simulink subsystem "mesh_assembly"  (R2021a)
settings: Solver=VariableStepAuto  StartTime=0.0  StopTime=10.0  RelTol=1e-3
undefined symbols (not defined in the file): dnm, knm, X, Y, Z
libraries: sm_lib x110, mesh_assembly_library x15
(part 2 of 4)

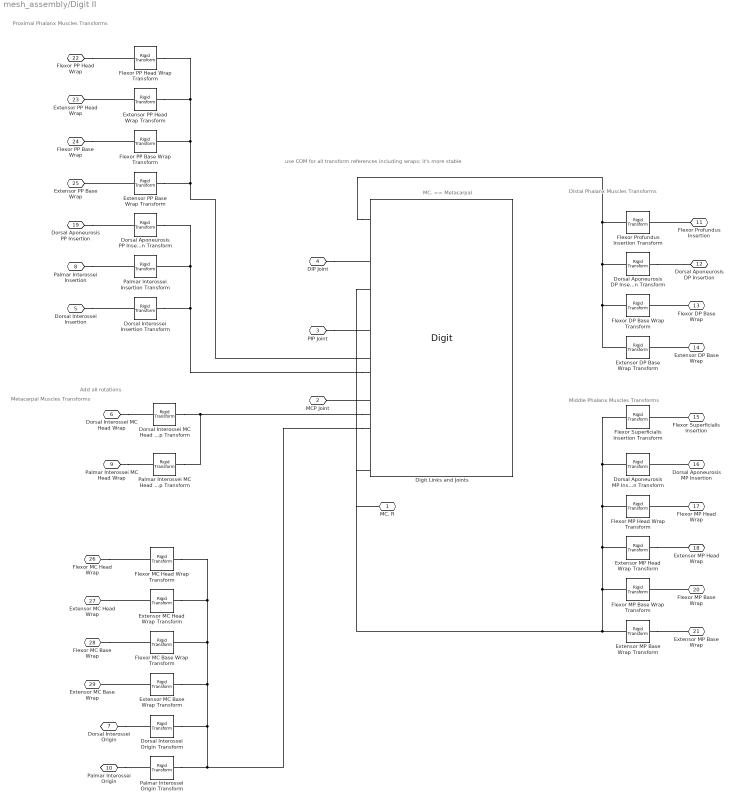
== system mesh_assembly/Digit II ==
  note: MC. == Metacarpal
  note: Proximal Phalanx Muscles Transforms
  note: Distal Phalanx Muscles Transforms
  note: Middle Phalanx Muscles Transforms
  note: Metacarpal Muscles Transforms
  note: Add all rotations
  note: use COM for all transform references including wraps: it's more stable
  Digit Links and Joints : mesh_assembly_library/Digit  links_density=dnm.link_density  distal_phalanx=knm.d2.distal_phalanx.file_name  distal_phalanx_base=knm.d2.distal_phalanx.base_transform  distal_phalanx_dip_joint=knm.d2.distal_phalanx.dip_joint_transform  distal_phalanx_head=knm.d2.distal_phalanx.head_transform  middle_phalanx=knm.d2.middle_phalanx.file_name  middle_phalanx_base=knm.d2.middle_phalanx.base_transform  middle_phalanx_pip_joint=knm.d2.middle_phalanx.pip_joint_transform  middle_phalanx_head=knm.d2.middle_phalanx.head_transform  middle_phalanx_dip_joint=knm.d2.middle_phalanx.dip_joint_transform  proximal_phalanx=knm.d2.proximal_phalanx.file_name  proximal_phalanx_base=knm.d2.proximal_phalanx.base_transform  proximal_phalanx_mcp_joint=knm.d2.proximal_phalanx.mcp_joint_transform  proximal_phalanx_head=knm.d2.proximal_phalanx.head_transform  proximal_phalanx_pip_joint=knm.d2.proximal_phalanx.pip_joint_transform  metacarpal=knm.d2.metacarpal.file_name  metacarpal_base=knm.d2.metacarpal.base_transform  metacarpal_cm_joint=knm.d2.metacarpal.cm_joint_transform  metacarpal_head=knm.d2.metacarpal.head_transform  metacarpal_mcp_joint=knm.d2.metacarpal.mcp_joint_transform  mcp_viz_radius=viz.d2.mcp_joint.radius  mcp_viz_color=viz.d2.mcp_joint.color  mcp_viz_opacity=viz.d2.mcp_joint.opacity  pip_viz_radius=viz.d2.pip_joint.radius  pip_viz_length=viz.d2.pip_joint.length  pip_viz_thickness=viz.d2.pip_joint.thickness  pip_viz_color=viz.d2.pip_joint.color  pip_viz_opacity=viz.d2.pip_joint.opacity  dip_viz_radius=viz.d2.dip_joint.radius  dip_viz_length=viz.d2.dip_joint.length  dip_viz_thickness=viz.d2.dip_joint.thickness  dip_viz_color=viz.d2.dip_joint.color  dip_viz_opacity=viz.d2.dip_joint.opacity
  Dorsal Aponeurosis DP Insertion Transform : sm_lib/Frames and Transforms/Rigid Transform  TranslationMethod=Cartesian  TranslationStandardOffset=0  TranslationLengthUnit=m  TranslationStandardAxis=+Z  TranslationCartesianOffset=knm.d2.distal_phalanx.dorsal_aponeurosis_DP_insertion(1,:)  TranslationROffset=0  TranslationROffsetUnits=m  TranslationZOffset=0  TranslationZOffsetUnits=m  TranslationThetaOffset=0  TranslationThetaOffsetUnits=deg  RotationMethod=RotationSequence  RotationAngleUnits=deg  RotationStandardAxis=+Z  RotationAngle=0.0  RotationArbitraryAxis=[0 0 1]  FollAlignAxisA=+X  BaseAlignAxisA=+Y  FollAlignAxisB=+Y  BaseAlignAxisB=+Z  RotationSequenceAxes=FollowerAxes  RotationSequence=XYZ  RotationSequenceAngles=knm.d2.distal_phalanx.dorsal_aponeurosis_DP_insertion(2,:)  RotationSequenceAnglesUnits=deg  RotationMatrix=[1 0 0; 0 1 0; 0 0 1]
  Dorsal Aponeurosis MP Insertion Transform : sm_lib/Frames and Transforms/Rigid Transform  TranslationMethod=Cartesian  TranslationStandardOffset=0  TranslationLengthUnit=m  TranslationStandardAxis=+Z  TranslationCartesianOffset=knm.d2.middle_phalanx.dorsal_aponeurosis_MP_insertion(1,:)  TranslationROffset=0  TranslationROffsetUnits=m  TranslationZOffset=0  TranslationZOffsetUnits=m  TranslationThetaOffset=0  TranslationThetaOffsetUnits=deg  RotationMethod=RotationSequence  RotationAngleUnits=deg  RotationStandardAxis=+Z  RotationAngle=0.0  RotationArbitraryAxis=[0 0 1]  FollAlignAxisA=+X  BaseAlignAxisA=+Y  FollAlignAxisB=+Y  BaseAlignAxisB=+Z  RotationSequenceAxes=FollowerAxes  RotationSequence=XYZ  RotationSequenceAngles=knm.d2.middle_phalanx.dorsal_aponeurosis_MP_insertion(2,:)  RotationSequenceAnglesUnits=deg  RotationMatrix=[1 0 0; 0 1 0; 0 0 1]
  Dorsal Aponeurosis PP Insertion Transform : sm_lib/Frames and Transforms/Rigid Transform  TranslationMethod=Cartesian  TranslationStandardOffset=0  TranslationLengthUnit=m  TranslationStandardAxis=+Z  TranslationCartesianOffset=knm.d2.proximal_phalanx.dorsal_aponeurosis_PP_insertion(1,:)  TranslationROffset=0  TranslationROffsetUnits=m  TranslationZOffset=0  TranslationZOffsetUnits=m  TranslationThetaOffset=0  TranslationThetaOffsetUnits=deg  RotationMethod=RotationSequence  RotationAngleUnits=deg  RotationStandardAxis=+Z  RotationAngle=0.0  RotationArbitraryAxis=[0 0 1]  FollAlignAxisA=+X  BaseAlignAxisA=+Y  FollAlignAxisB=+Y  BaseAlignAxisB=+Z  RotationSequenceAxes=FollowerAxes  RotationSequence=XYZ  RotationSequenceAngles=knm.d2.proximal_phalanx.dorsal_aponeurosis_PP_insertion(2,:)  RotationSequenceAnglesUnits=deg  RotationMatrix=[1 0 0; 0 1 0; 0 0 1]
  Dorsal Interossei Insertion Transform : sm_lib/Frames and Transforms/Rigid Transform  TranslationMethod=Cartesian  TranslationStandardOffset=0  TranslationLengthUnit=m  TranslationStandardAxis=+Z  TranslationCartesianOffset=knm.d2.proximal_phalanx.dorsal_interossei_insertion_point_transform(1,:)  TranslationROffset=0  TranslationROffsetUnits=m  TranslationZOffset=0  TranslationZOffsetUnits=m  TranslationThetaOffset=0  TranslationThetaOffsetUnits=deg  RotationMethod=RotationSequence  RotationAngleUnits=deg  RotationStandardAxis=+Z  RotationAngle=0.0  RotationArbitraryAxis=[0 0 1]  FollAlignAxisA=+X  BaseAlignAxisA=+Y  FollAlignAxisB=+Y  BaseAlignAxisB=+Z  RotationSequenceAxes=FollowerAxes  RotationSequence=XYZ  RotationSequenceAngles=knm.d2.proximal_phalanx.dorsal_interossei_insertion_point_transform(2,:)  RotationSequenceAnglesUnits=deg  RotationMatrix=[1 0 0; 0 1 0; 0 0 1]
  Dorsal Interossei MC Head Wrap Transform : sm_lib/Frames and Transforms/Rigid Transform  TranslationMethod=Cartesian  TranslationStandardOffset=0  TranslationLengthUnit=m  TranslationStandardAxis=+Z  TranslationCartesianOffset=knm.d2.metacarpal.dorsal_interossei_mc_head_wrap_transform(1,:)  TranslationROffset=0  TranslationROffsetUnits=m  TranslationZOffset=0  TranslationZOffsetUnits=m  TranslationThetaOffset=0  TranslationThetaOffsetUnits=deg  RotationMethod=RotationSequence  RotationAngleUnits=deg  RotationStandardAxis=+Z  RotationAngle=0.0  RotationArbitraryAxis=[0 0 1]  FollAlignAxisA=+X  BaseAlignAxisA=+Y  FollAlignAxisB=+Y  BaseAlignAxisB=+Z  RotationSequenceAxes=FollowerAxes  RotationSequence=XYZ  RotationSequenceAngles=knm.d2.metacarpal.dorsal_interossei_mc_head_wrap_transform(2,:)  RotationSequenceAnglesUnits=deg  RotationMatrix=[1 0 0; 0 1 0; 0 0 1]
  Dorsal Interossei Origin Transform : sm_lib/Frames and Transforms/Rigid Transform  TranslationMethod=Cartesian  TranslationStandardOffset=0  TranslationLengthUnit=m  TranslationStandardAxis=+Z  TranslationCartesianOffset=knm.d2.metacarpal.dorsal_interossei_origin_point_transform(1,:)  TranslationROffset=0  TranslationROffsetUnits=m  TranslationZOffset=0  TranslationZOffsetUnits=m  TranslationThetaOffset=0  TranslationThetaOffsetUnits=deg  RotationMethod=RotationSequence  RotationAngleUnits=deg  RotationStandardAxis=+Z  RotationAngle=0.0  RotationArbitraryAxis=[0 0 1]  FollAlignAxisA=+X  BaseAlignAxisA=+Y  FollAlignAxisB=+Y  BaseAlignAxisB=+Z  RotationSequenceAxes=FollowerAxes  RotationSequence=XYZ  RotationSequenceAngles=knm.d2.metacarpal.dorsal_interossei_origin_point_transform(2,:)  RotationSequenceAnglesUnits=deg  RotationMatrix=[1 0 0; 0 1 0; 0 0 1]
  Extensor DP Base Wrap Transform : sm_lib/Frames and Transforms/Rigid Transform  TranslationMethod=Cartesian  TranslationStandardOffset=0  TranslationLengthUnit=m  TranslationStandardAxis=+Z  TranslationCartesianOffset=knm.d2.distal_phalanx.extensor_base_wrap(1,:)  TranslationROffset=0  TranslationROffsetUnits=m  TranslationZOffset=0  TranslationZOffsetUnits=m  TranslationThetaOffset=0  TranslationThetaOffsetUnits=deg  RotationMethod=RotationSequence  RotationAngleUnits=deg  RotationStandardAxis=+Z  RotationAngle=0.0  RotationArbitraryAxis=[0 0 1]  FollAlignAxisA=+X  BaseAlignAxisA=+Y  FollAlignAxisB=+Y  BaseAlignAxisB=+Z  RotationSequenceAxes=FollowerAxes  RotationSequence=XYZ  RotationSequenceAngles=knm.d2.distal_phalanx.extensor_base_wrap(2,:)  RotationSequenceAnglesUnits=deg  RotationMatrix=[1 0 0; 0 1 0; 0 0 1]
  Extensor MC Base Wrap Transform : sm_lib/Frames and Transforms/Rigid Transform  TranslationMethod=Cartesian  TranslationStandardOffset=0  TranslationLengthUnit=m  TranslationStandardAxis=+Z  TranslationCartesianOffset=knm.d2.metacarpal.extensor_base_wrap(1,:)  TranslationROffset=0  TranslationROffsetUnits=m  TranslationZOffset=0  TranslationZOffsetUnits=m  TranslationThetaOffset=0  TranslationThetaOffsetUnits=deg  RotationMethod=RotationSequence  RotationAngleUnits=deg  RotationStandardAxis=+Z  RotationAngle=0.0  RotationArbitraryAxis=[0 0 1]  FollAlignAxisA=+X  BaseAlignAxisA=+Y  FollAlignAxisB=+Y  BaseAlignAxisB=+Z  RotationSequenceAxes=FollowerAxes  RotationSequence=XYZ  RotationSequenceAngles=knm.d2.metacarpal.extensor_base_wrap(2,:)  RotationSequenceAnglesUnits=deg  RotationMatrix=[1 0 0; 0 1 0; 0 0 1]
  Extensor MC Head Wrap Transform : sm_lib/Frames and Transforms/Rigid Transform  TranslationMethod=Cartesian  TranslationStandardOffset=0  TranslationLengthUnit=m  TranslationStandardAxis=+Z  TranslationCartesianOffset=knm.d2.metacarpal.extensor_head_wrap(1,:)  TranslationROffset=0  TranslationROffsetUnits=m  TranslationZOffset=0  TranslationZOffsetUnits=m  TranslationThetaOffset=0  TranslationThetaOffsetUnits=deg  RotationMethod=RotationSequence  RotationAngleUnits=deg  RotationStandardAxis=+Z  RotationAngle=0.0  RotationArbitraryAxis=[0 0 1]  FollAlignAxisA=+X  BaseAlignAxisA=+Y  FollAlignAxisB=+Y  BaseAlignAxisB=+Z  RotationSequenceAxes=FollowerAxes  RotationSequence=XYZ  RotationSequenceAngles=knm.d2.metacarpal.extensor_head_wrap(2,:)  RotationSequenceAnglesUnits=deg  RotationMatrix=[1 0 0; 0 1 0; 0 0 1]
  Extensor MP Base Wrap Transform : sm_lib/Frames and Transforms/Rigid Transform  TranslationMethod=Cartesian  TranslationStandardOffset=0  TranslationLengthUnit=m  TranslationStandardAxis=+Z  TranslationCartesianOffset=knm.d2.middle_phalanx.extensor_base_wrap(1,:)  TranslationROffset=0  TranslationROffsetUnits=m  TranslationZOffset=0  TranslationZOffsetUnits=m  TranslationThetaOffset=0  TranslationThetaOffsetUnits=deg  RotationMethod=RotationSequence  RotationAngleUnits=deg  RotationStandardAxis=+Z  RotationAngle=0.0  RotationArbitraryAxis=[0 0 1]  FollAlignAxisA=+X  BaseAlignAxisA=+Y  FollAlignAxisB=+Y  BaseAlignAxisB=+Z  RotationSequenceAxes=FollowerAxes  RotationSequence=XYZ  RotationSequenceAngles=knm.d2.middle_phalanx.extensor_base_wrap(2,:)  RotationSequenceAnglesUnits=deg  RotationMatrix=[1 0 0; 0 1 0; 0 0 1]
  Extensor MP Head Wrap Transform : sm_lib/Frames and Transforms/Rigid Transform  TranslationMethod=Cartesian  TranslationStandardOffset=0  TranslationLengthUnit=m  TranslationStandardAxis=+Z  TranslationCartesianOffset=knm.d2.middle_phalanx.extensor_head_wrap(1,:)  TranslationROffset=0  TranslationROffsetUnits=m  TranslationZOffset=0  TranslationZOffsetUnits=m  TranslationThetaOffset=0  TranslationThetaOffsetUnits=deg  RotationMethod=RotationSequence  RotationAngleUnits=deg  RotationStandardAxis=+Z  RotationAngle=0.0  RotationArbitraryAxis=[0 0 1]  FollAlignAxisA=+X  BaseAlignAxisA=+Y  FollAlignAxisB=+Y  BaseAlignAxisB=+Z  RotationSequenceAxes=FollowerAxes  RotationSequence=XYZ  RotationSequenceAngles=knm.d2.middle_phalanx.extensor_head_wrap(2,:)  RotationSequenceAnglesUnits=deg  RotationMatrix=[1 0 0; 0 1 0; 0 0 1]
  Extensor PP Base Wrap Transform : sm_lib/Frames and Transforms/Rigid Transform  TranslationMethod=Cartesian  TranslationStandardOffset=0  TranslationLengthUnit=m  TranslationStandardAxis=+Z  TranslationCartesianOffset=knm.d2.proximal_phalanx.extensor_base_wrap(1,:)  TranslationROffset=0  TranslationROffsetUnits=m  TranslationZOffset=0  TranslationZOffsetUnits=m  TranslationThetaOffset=0  TranslationThetaOffsetUnits=deg  RotationMethod=RotationSequence  RotationAngleUnits=deg  RotationStandardAxis=+Z  RotationAngle=0.0  RotationArbitraryAxis=[0 0 1]  FollAlignAxisA=+X  BaseAlignAxisA=+Y  FollAlignAxisB=+Y  BaseAlignAxisB=+Z  RotationSequenceAxes=FollowerAxes  RotationSequence=XYZ  RotationSequenceAngles=knm.d2.proximal_phalanx.extensor_base_wrap(2,:)  RotationSequenceAnglesUnits=deg  RotationMatrix=[1 0 0; 0 1 0; 0 0 1]
  Extensor PP Head Wrap Transform : sm_lib/Frames and Transforms/Rigid Transform  TranslationMethod=Cartesian  TranslationStandardOffset=0  TranslationLengthUnit=m  TranslationStandardAxis=+Z  TranslationCartesianOffset=knm.d2.proximal_phalanx.extensor_head_wrap(1,:)  TranslationROffset=0  TranslationROffsetUnits=m  TranslationZOffset=0  TranslationZOffsetUnits=m  TranslationThetaOffset=0  TranslationThetaOffsetUnits=deg  RotationMethod=RotationSequence  RotationAngleUnits=deg  RotationStandardAxis=+Z  RotationAngle=0.0  RotationArbitraryAxis=[0 0 1]  FollAlignAxisA=+X  BaseAlignAxisA=+Y  FollAlignAxisB=+Y  BaseAlignAxisB=+Z  RotationSequenceAxes=FollowerAxes  RotationSequence=XYZ  RotationSequenceAngles=knm.d2.proximal_phalanx.extensor_head_wrap(2,:)  RotationSequenceAnglesUnits=deg  RotationMatrix=[1 0 0; 0 1 0; 0 0 1]
  Flexor DP Base Wrap Transform : sm_lib/Frames and Transforms/Rigid Transform  TranslationMethod=Cartesian  TranslationStandardOffset=0  TranslationLengthUnit=m  TranslationStandardAxis=+Z  TranslationCartesianOffset=knm.d2.distal_phalanx.flexor_base_wrap(1,:)  TranslationROffset=0  TranslationROffsetUnits=m  TranslationZOffset=0  TranslationZOffsetUnits=m  TranslationThetaOffset=0  TranslationThetaOffsetUnits=deg  RotationMethod=RotationSequence  RotationAngleUnits=deg  RotationStandardAxis=+Z  RotationAngle=0.0  RotationArbitraryAxis=[0 0 1]  FollAlignAxisA=+X  BaseAlignAxisA=+Y  FollAlignAxisB=+Y  BaseAlignAxisB=+Z  RotationSequenceAxes=FollowerAxes  RotationSequence=XYZ  RotationSequenceAngles=knm.d2.distal_phalanx.flexor_base_wrap(2,:)  RotationSequenceAnglesUnits=deg  RotationMatrix=[1 0 0; 0 1 0; 0 0 1]
  Flexor MC Base Wrap Transform : sm_lib/Frames and Transforms/Rigid Transform  TranslationMethod=Cartesian  TranslationStandardOffset=0  TranslationLengthUnit=m  TranslationStandardAxis=+Z  TranslationCartesianOffset=knm.d2.metacarpal.flexor_base_wrap(1,:)  TranslationROffset=0  TranslationROffsetUnits=m  TranslationZOffset=0  TranslationZOffsetUnits=m  TranslationThetaOffset=0  TranslationThetaOffsetUnits=deg  RotationMethod=RotationSequence  RotationAngleUnits=deg  RotationStandardAxis=+Z  RotationAngle=0.0  RotationArbitraryAxis=[0 0 1]  FollAlignAxisA=+X  BaseAlignAxisA=+Y  FollAlignAxisB=+Y  BaseAlignAxisB=+Z  RotationSequenceAxes=FollowerAxes  RotationSequence=XYZ  RotationSequenceAngles=knm.d2.metacarpal.flexor_base_wrap(2,:)  RotationSequenceAnglesUnits=deg  RotationMatrix=[1 0 0; 0 1 0; 0 0 1]
  Flexor MC Head Wrap Transform : sm_lib/Frames and Transforms/Rigid Transform  TranslationMethod=Cartesian  TranslationStandardOffset=0  TranslationLengthUnit=m  TranslationStandardAxis=+Z  TranslationCartesianOffset=knm.d2.metacarpal.flexor_head_wrap(1,:)  TranslationROffset=0  TranslationROffsetUnits=m  TranslationZOffset=0  TranslationZOffsetUnits=m  TranslationThetaOffset=0  TranslationThetaOffsetUnits=deg  RotationMethod=RotationSequence  RotationAngleUnits=deg  RotationStandardAxis=+Z  RotationAngle=0.0  RotationArbitraryAxis=[0 0 1]  FollAlignAxisA=+X  BaseAlignAxisA=+Y  FollAlignAxisB=+Y  BaseAlignAxisB=+Z  RotationSequenceAxes=FollowerAxes  RotationSequence=XYZ  RotationSequenceAngles=knm.d2.metacarpal.flexor_head_wrap(2,:)  RotationSequenceAnglesUnits=deg  RotationMatrix=[1 0 0; 0 1 0; 0 0 1]
  Flexor MP Base Wrap Transform : sm_lib/Frames and Transforms/Rigid Transform  TranslationMethod=Cartesian  TranslationStandardOffset=0  TranslationLengthUnit=m  TranslationStandardAxis=+Z  TranslationCartesianOffset=knm.d2.middle_phalanx.flexor_base_wrap(1,:)  TranslationROffset=0  TranslationROffsetUnits=m  TranslationZOffset=0  TranslationZOffsetUnits=m  TranslationThetaOffset=0  TranslationThetaOffsetUnits=deg  RotationMethod=RotationSequence  RotationAngleUnits=deg  RotationStandardAxis=+Z  RotationAngle=0.0  RotationArbitraryAxis=[0 0 1]  FollAlignAxisA=+X  BaseAlignAxisA=+Y  FollAlignAxisB=+Y  BaseAlignAxisB=+Z  RotationSequenceAxes=FollowerAxes  RotationSequence=XYZ  RotationSequenceAngles=knm.d2.middle_phalanx.flexor_base_wrap(2,:)  RotationSequenceAnglesUnits=deg  RotationMatrix=[1 0 0; 0 1 0; 0 0 1]
  Flexor MP Head Wrap Transform : sm_lib/Frames and Transforms/Rigid Transform  TranslationMethod=Cartesian  TranslationStandardOffset=0  TranslationLengthUnit=m  TranslationStandardAxis=+Z  TranslationCartesianOffset=knm.d2.middle_phalanx.flexor_head_wrap(1,:)  TranslationROffset=0  TranslationROffsetUnits=m  TranslationZOffset=0  TranslationZOffsetUnits=m  TranslationThetaOffset=0  TranslationThetaOffsetUnits=deg  RotationMethod=RotationSequence  RotationAngleUnits=deg  RotationStandardAxis=+Z  RotationAngle=0.0  RotationArbitraryAxis=[0 0 1]  FollAlignAxisA=+X  BaseAlignAxisA=+Y  FollAlignAxisB=+Y  BaseAlignAxisB=+Z  RotationSequenceAxes=FollowerAxes  RotationSequence=XYZ  RotationSequenceAngles=knm.d2.middle_phalanx.flexor_head_wrap(2,:)  RotationSequenceAnglesUnits=deg  RotationMatrix=[1 0 0; 0 1 0; 0 0 1]
  Flexor PP Base Wrap Transform : sm_lib/Frames and Transforms/Rigid Transform  TranslationMethod=Cartesian  TranslationStandardOffset=0  TranslationLengthUnit=m  TranslationStandardAxis=+Z  TranslationCartesianOffset=knm.d2.proximal_phalanx.flexor_base_wrap(1,:)  TranslationROffset=0  TranslationROffsetUnits=m  TranslationZOffset=0  TranslationZOffsetUnits=m  TranslationThetaOffset=0  TranslationThetaOffsetUnits=deg  RotationMethod=RotationSequence  RotationAngleUnits=deg  RotationStandardAxis=+Z  RotationAngle=0.0  RotationArbitraryAxis=[0 0 1]  FollAlignAxisA=+X  BaseAlignAxisA=+Y  FollAlignAxisB=+Y  BaseAlignAxisB=+Z  RotationSequenceAxes=FollowerAxes  RotationSequence=XYZ  RotationSequenceAngles=knm.d2.proximal_phalanx.flexor_base_wrap(2,:)  RotationSequenceAnglesUnits=deg  RotationMatrix=[1 0 0; 0 1 0; 0 0 1]
  Flexor PP Head Wrap Transform : sm_lib/Frames and Transforms/Rigid Transform  TranslationMethod=Cartesian  TranslationStandardOffset=0  TranslationLengthUnit=m  TranslationStandardAxis=+Z  TranslationCartesianOffset=knm.d2.proximal_phalanx.flexor_head_wrap(1,:)  TranslationROffset=0  TranslationROffsetUnits=m  TranslationZOffset=0  TranslationZOffsetUnits=m  TranslationThetaOffset=0  TranslationThetaOffsetUnits=deg  RotationMethod=RotationSequence  RotationAngleUnits=deg  RotationStandardAxis=+Z  RotationAngle=0.0  RotationArbitraryAxis=[0 0 1]  FollAlignAxisA=+X  BaseAlignAxisA=+Y  FollAlignAxisB=+Y  BaseAlignAxisB=+Z  RotationSequenceAxes=FollowerAxes  RotationSequence=XYZ  RotationSequenceAngles=knm.d2.proximal_phalanx.flexor_head_wrap(2,:)  RotationSequenceAnglesUnits=deg  RotationMatrix=[1 0 0; 0 1 0; 0 0 1]
  Flexor Profundus Insertion Transform : sm_lib/Frames and Transforms/Rigid Transform  TranslationMethod=Cartesian  TranslationStandardOffset=0  TranslationLengthUnit=m  TranslationStandardAxis=+Z  TranslationCartesianOffset=knm.d2.distal_phalanx.flexor_profundus_insertion(1,:)  TranslationROffset=0  TranslationROffsetUnits=m  TranslationZOffset=0  TranslationZOffsetUnits=m  TranslationThetaOffset=0  TranslationThetaOffsetUnits=deg  RotationMethod=RotationSequence  RotationAngleUnits=deg  RotationStandardAxis=+Z  RotationAngle=0.0  RotationArbitraryAxis=[0 0 1]  FollAlignAxisA=+X  BaseAlignAxisA=+Y  FollAlignAxisB=+Y  BaseAlignAxisB=+Z  RotationSequenceAxes=FollowerAxes  RotationSequence=XYZ  RotationSequenceAngles=knm.d2.distal_phalanx.flexor_profundus_insertion(2,:)  RotationSequenceAnglesUnits=deg  RotationMatrix=[1 0 0; 0 1 0; 0 0 1]
  Flexor Superficialis Insertion Transform : sm_lib/Frames and Transforms/Rigid Transform  TranslationMethod=Cartesian  TranslationStandardOffset=0  TranslationLengthUnit=m  TranslationStandardAxis=+Z  TranslationCartesianOffset=knm.d2.middle_phalanx.flexor_superficialis_insertion(1,:)  TranslationROffset=0  TranslationROffsetUnits=m  TranslationZOffset=0  TranslationZOffsetUnits=m  TranslationThetaOffset=0  TranslationThetaOffsetUnits=deg  RotationMethod=RotationSequence  RotationAngleUnits=deg  RotationStandardAxis=+Z  RotationAngle=0.0  RotationArbitraryAxis=[0 0 1]  FollAlignAxisA=+X  BaseAlignAxisA=+Y  FollAlignAxisB=+Y  BaseAlignAxisB=+Z  RotationSequenceAxes=FollowerAxes  RotationSequence=XYZ  RotationSequenceAngles=knm.d2.middle_phalanx.flexor_superficialis_insertion(2,:)  RotationSequenceAnglesUnits=deg  RotationMatrix=[1 0 0; 0 1 0; 0 0 1]
  Palmar Interossei Insertion Transform : sm_lib/Frames and Transforms/Rigid Transform  TranslationMethod=Cartesian  TranslationStandardOffset=0  TranslationLengthUnit=m  TranslationStandardAxis=+Z  TranslationCartesianOffset=knm.d2.proximal_phalanx.palmar_interossei_insertion_point_transform(1,:)  TranslationROffset=0  TranslationROffsetUnits=m  TranslationZOffset=0  TranslationZOffsetUnits=m  TranslationThetaOffset=0  TranslationThetaOffsetUnits=deg  RotationMethod=RotationSequence  RotationAngleUnits=deg  RotationStandardAxis=+Z  RotationAngle=0.0  RotationArbitraryAxis=[0 0 1]  FollAlignAxisA=+X  BaseAlignAxisA=+Y  FollAlignAxisB=+Y  BaseAlignAxisB=+Z  RotationSequenceAxes=FollowerAxes  RotationSequence=XYZ  RotationSequenceAngles=knm.d2.proximal_phalanx.palmar_interossei_insertion_point_transform(2,:)  RotationSequenceAnglesUnits=deg  RotationMatrix=[1 0 0; 0 1 0; 0 0 1]
  Palmar Interossei MC Head Wrap Transform : sm_lib/Frames and Transforms/Rigid Transform  TranslationMethod=Cartesian  TranslationStandardOffset=0  TranslationLengthUnit=m  TranslationStandardAxis=+Z  TranslationCartesianOffset=knm.d2.metacarpal.palmar_interossei_mc_head_wrap_transform(1,:)  TranslationROffset=0  TranslationROffsetUnits=m  TranslationZOffset=0  TranslationZOffsetUnits=m  TranslationThetaOffset=0  TranslationThetaOffsetUnits=deg  RotationMethod=RotationSequence  RotationAngleUnits=deg  RotationStandardAxis=+Z  RotationAngle=0.0  RotationArbitraryAxis=[0 0 1]  FollAlignAxisA=+X  BaseAlignAxisA=+Y  FollAlignAxisB=+Y  BaseAlignAxisB=+Z  RotationSequenceAxes=FollowerAxes  RotationSequence=XYZ  RotationSequenceAngles=knm.d2.metacarpal.palmar_interossei_mc_head_wrap_transform(2,:)  RotationSequenceAnglesUnits=deg  RotationMatrix=[1 0 0; 0 1 0; 0 0 1]
  Palmar Interossei Origin Transform : sm_lib/Frames and Transforms/Rigid Transform  TranslationMethod=Cartesian  TranslationStandardOffset=0  TranslationLengthUnit=m  TranslationStandardAxis=+Z  TranslationCartesianOffset=knm.d2.metacarpal.palmar_interossei_origin_point_transform(1,:)  TranslationROffset=0  TranslationROffsetUnits=m  TranslationZOffset=0  TranslationZOffsetUnits=m  TranslationThetaOffset=0  TranslationThetaOffsetUnits=deg  RotationMethod=RotationSequence  RotationAngleUnits=deg  RotationStandardAxis=+Z  RotationAngle=0.0  RotationArbitraryAxis=[0 0 1]  FollAlignAxisA=+X  BaseAlignAxisA=+Y  FollAlignAxisB=+Y  BaseAlignAxisB=+Z  RotationSequenceAxes=FollowerAxes  RotationSequence=XYZ  RotationSequenceAngles=knm.d2.metacarpal.palmar_interossei_origin_point_transform(2,:)  RotationSequenceAnglesUnits=deg  RotationMatrix=[1 0 0; 0 1 0; 0 0 1]
  MC. R : PMIOPort  Side=Left
  MCP Joint : PMIOPort  Port=2  Side=Left
  PIP Joint : PMIOPort  Port=3  Side=Left
  DIP Joint : PMIOPort  Port=4  Side=Left
  Dorsal Interossei Insertion : PMIOPort  Port=5  Side=Left
  Dorsal Interossei MC Head Wrap : PMIOPort  Port=6  Side=Left
  Dorsal Interossei Origin : PMIOPort  Port=7  Side=Left
  Palmar Interossei Insertion : PMIOPort  Port=8  Side=Left
  Palmar Interossei MC Head Wrap : PMIOPort  Port=9  Side=Left
  Palmar Interossei Origin : PMIOPort  Port=10  Side=Left
  Flexor Profundus Insertion : PMIOPort  Port=11  Side=Left
  Dorsal Aponeurosis DP Insertion : PMIOPort  Port=12  Side=Left
  Flexor DP Base Wrap : PMIOPort  Port=13  Side=Left
  Extensor DP Base Wrap : PMIOPort  Port=14  Side=Left
  Flexor Superficialis Insertion : PMIOPort  Port=15  Side=Left
  Dorsal Aponeurosis MP Insertion : PMIOPort  Port=16  Side=Left
  Flexor MP Head Wrap : PMIOPort  Port=17  Side=Left
  Extensor MP Head Wrap : PMIOPort  Port=18  Side=Left
  Dorsal Aponeurosis PP Insertion : PMIOPort  Port=19  Side=Left
  Flexor MP Base Wrap : PMIOPort  Port=20  Side=Left
  Extensor MP Base Wrap : PMIOPort  Port=21  Side=Left
  Flexor PP Head Wrap : PMIOPort  Port=22  Side=Left
  Extensor PP Head Wrap : PMIOPort  Port=23  Side=Left
  Flexor PP Base Wrap : PMIOPort  Port=24  Side=Left
  Extensor PP Base Wrap : PMIOPort  Port=25  Side=Left
  Flexor MC Head Wrap : PMIOPort  Port=26  Side=Left
  Extensor MC Head Wrap : PMIOPort  Port=27  Side=Left
  Flexor MC Base Wrap : PMIOPort  Port=28  Side=Left
  Extensor MC Base Wrap : PMIOPort  Port=29  Side=Left
  connections:
  Extensor MC Base Wrap Transform/RConn1 -- Extensor MC Base Wrap/RConn1
  Flexor MC Base Wrap/RConn1 -- Flexor MC Base Wrap Transform/RConn1
  Flexor MC Head Wrap/RConn1 -- Flexor MC Head Wrap Transform/RConn1
  Extensor MC Head Wrap Transform/RConn1 -- Extensor MC Head Wrap/RConn1
  Digit Links and Joints/LConn17 -- Palmar Interossei Origin Transform/LConn1 -- Dorsal Interossei Origin Transform/LConn1 -- Extensor MC Base Wrap Transform/LConn1 -- Flexor MC Head Wrap Transform/LConn1 -- Extensor MC Head Wrap Transform/LConn1 -- Flexor MC Base Wrap Transform/LConn1
  Digit Links and Joints/LConn12 -- Extensor PP Base Wrap Transform/LConn1 -- Flexor PP Base Wrap Transform/LConn1 -- Extensor PP Head Wrap Transform/LConn1 -- Flexor PP Head Wrap Transform/LConn1
  Extensor PP Head Wrap Transform/RConn1 -- Extensor PP Head Wrap/RConn1
  Flexor PP Head Wrap/RConn1 -- Flexor PP Head Wrap Transform/RConn1
  Flexor PP Base Wrap/RConn1 -- Flexor PP Base Wrap Transform/RConn1
  Extensor PP Base Wrap Transform/RConn1 -- Extensor PP Base Wrap/RConn1
  Digit Links and Joints/LConn13 -- Palmar Interossei Insertion Transform/LConn1 -- Dorsal Aponeurosis PP Insertion Transform/LConn1 -- Dorsal Interossei Insertion Transform/LConn1
  Flexor MP Base Wrap/RConn1 -- Flexor MP Base Wrap Transform/RConn1
  Extensor MP Base Wrap Transform/RConn1 -- Extensor MP Base Wrap/RConn1
  Dorsal Aponeurosis PP Insertion/RConn1 -- Dorsal Aponeurosis PP Insertion Transform/RConn1
  Extensor MP Head Wrap Transform/RConn1 -- Extensor MP Head Wrap/RConn1
  Flexor MP Head Wrap/RConn1 -- Flexor MP Head Wrap Transform/RConn1
  Dorsal Aponeurosis MP Insertion/RConn1 -- Dorsal Aponeurosis MP Insertion Transform/RConn1
  Flexor Superficialis Insertion/RConn1 -- Flexor Superficialis Insertion Transform/RConn1
  Dorsal Aponeurosis DP Insertion Transform/RConn1 -- Dorsal Aponeurosis DP Insertion/RConn1
  Flexor DP Base Wrap/RConn1 -- Flexor DP Base Wrap Transform/RConn1
  Extensor DP Base Wrap/RConn1 -- Extensor DP Base Wrap Transform/RConn1
  Flexor Profundus Insertion/RConn1 -- Flexor Profundus Insertion Transform/RConn1
  Digit Links and Joints/LConn2 -- Dorsal Aponeurosis DP Insertion Transform/LConn1 -- Flexor DP Base Wrap Transform/LConn1 -- Extensor DP Base Wrap Transform/LConn1 -- Flexor Profundus Insertion Transform/LConn1
  Digit Links and Joints/LConn7 -- Extensor MP Base Wrap Transform/LConn1 -- Flexor MP Base Wrap Transform/LConn1 -- Extensor MP Head Wrap Transform/LConn1 -- Flexor MP Head Wrap Transform/LConn1 -- Dorsal Aponeurosis MP Insertion Transform/LConn1 -- Flexor Superficialis Insertion Transform/LConn1
  Palmar Interossei Insertion/RConn1 -- Palmar Interossei Insertion Transform/RConn1
  Palmar Interossei MC Head Wrap/RConn1 -- Palmar Interossei MC Head Wrap Transform/RConn1
  Palmar Interossei Origin/RConn1 -- Palmar Interossei Origin Transform/RConn1
  Dorsal Interossei Origin/RConn1 -- Dorsal Interossei Origin Transform/RConn1
  Dorsal Interossei MC Head Wrap/RConn1 -- Dorsal Interossei MC Head Wrap Transform/RConn1
  Dorsal Interossei Insertion/RConn1 -- Dorsal Interossei Insertion Transform/RConn1
  Digit Links and Joints/LConn16 -- Dorsal Interossei MC Head Wrap Transform/LConn1 -- Palmar Interossei MC Head Wrap Transform/LConn1
  DIP Joint/RConn1 -- Digit Links and Joints/LConn5
  PIP Joint/RConn1 -- Digit Links and Joints/LConn10
  Digit Links and Joints/LConn15 -- MCP Joint/RConn1
  MC. R/RConn1 -- Digit Links and Joints/LConn20

== system mesh_assembly/Digit III ==
  note: MC. == Metacarpal
  Digit Links and Joints : Subsystem  AncestorBlock=mechanics_model_library/Digit  mask{links_density=dnm.link_density, distal_phalanx=knm.d3.distal_phalanx.file_name, distal_phalanx_base=knm.d3.distal_phalanx.base_transform, distal_phalanx_dip_joint=knm.d3.distal_phalanx.dip_joint_transform, distal_phalanx_head=knm.d3.distal_phalanx.head_transform, middle_phalanx=knm.d3.middle_phalanx.file_name, middle_phalanx_base=knm.d3.middle_phalanx.base_transform, middle_phalanx_pip_joint=knm.d3.middle_phalanx.pip_joint_transform, middle_phalanx_head=knm.d3.middle_phalanx.head_transform, middle_phalanx_dip_joint=knm.d3.middle_phalanx.dip_joint_transform, proximal_phalanx=knm.d3.proximal_phalanx.file_name, proximal_phalanx_base=knm.d3.proximal_phalanx.base_transform, proximal_phalanx_mcp_joint=knm.d3.proximal_phalanx.mcp_joint_transform, proximal_phalanx_head=knm.d3.proximal_phalanx.head_transform, proximal_phalanx_pip_joint=knm.d3.proximal_phalanx.pip_joint_transform, metacarpal=knm.d3.metacarpal.file_name, metacarpal_base=knm.d3.metacarpal.base_transform, metacarpal_cm_joint=knm.d3.metacarpal.cm_joint_transform, metacarpal_head=knm.d3.metacarpal.head_transform, metacarpal_mcp_joint=knm.d3.metacarpal.mcp_joint_transform, mcp_viz_radius=viz.d3.mcp_joint.radius, mcp_viz_color=viz.d3.mcp_joint.color, mcp_viz_opacity=viz.d3.mcp_joint.opacity, pip_viz_radius=viz.d3.pip_joint.radius, pip_viz_length=viz.d3.pip_joint.length, pip_viz_thickness=viz.d3.pip_joint.thickness, pip_viz_color=viz.d3.pip_joint.color, pip_viz_opacity=viz.d3.pip_joint.opacity, dip_viz_radius=viz.d3.dip_joint.radius, dip_viz_length=viz.d3.dip_joint.length, dip_viz_thickness=viz.d3.dip_joint.thickness, dip_viz_color=viz.d3.dip_joint.color, dip_viz_opacity=viz.d3.dip_joint.opacity}
      mask prompts: links_density "Density [Kg/(m^3)]"; distal_phalanx "File Name"; distal_phalanx_base "Base Transform (Translation [m], Rotation: X-Y-Z [deg])"; distal_phalanx_dip_joint "DIP Joint Transform (Translation, Rotation)"; distal_phalanx_head "Head Transform (Translation, Rotation)"; middle_phalanx "File Name"; middle_phalanx_base "Base Transform"; middle_phalanx_pip_joint "PIP Joint Transform"; middle_phalanx_head "Head Transform"; middle_phalanx_dip_joint "DIP Joint Transform"; proximal_phalanx "File Name"; proximal_phalanx_base "Base Transform"; proximal_phalanx_mcp_joint "MCP Joint Transform"; proximal_phalanx_head "Head Transform"; proximal_phalanx_pip_joint "PIP Joint Transform"; metacarpal "File Name"; metacarpal_base "Base Transform"; metacarpal_cm_joint "CM Joint Transform"; metacarpal_head "Head Transform"; metacarpal_mcp_joint "MCP Joint Transform"; mcp_viz_radius "Radius [m]"; mcp_viz_color "Color (RGB - Range [0, 1])"; mcp_viz_opacity "Opacity (Range [0, 1])"; pip_viz_radius "Radius [m]"; pip_viz_length "Length [m]"; pip_viz_thickness "Thickness [m]"; pip_viz_color "Color (RGB - Range [0, 1])"; pip_viz_opacity "Opacity (Range [0, 1])"; dip_viz_radius "Radius [m]"; dip_viz_length "Length [m]"; dip_viz_thickness "Thickness [m]"; dip_viz_color "Color (RGB - Range [0, 1])"; dip_viz_opacity "Opacity (Range [0, 1])"
      mask DialogControl DescGroupVar Prompt: Digit Subsystem
      mask DialogControl DescTextVar Prompt: This subsystem encapsulates the bones and joints that makes up digits II - V. Metacarpal bone, Proximal, Middle and Distal Phalanxes; MCP, PIP and DIP Joints.
      mask DialogControl Links Prompt: Links
      mask DialogControl Distal_Phalanx Prompt: Distal Phalanx
      mask DialogControl Middle_Phalanx Prompt: Middle Phalanx
      mask DialogControl Proximal_Phalanx Prompt: Proximal Phalanx
      mask DialogControl Metacarpal Prompt: Metacarpal
      mask DialogControl Container10 Prompt: Visualization
      mask DialogControl Container11 Prompt: MCP Joint
      mask DialogControl Container12 Prompt: PIP Joint
      mask DialogControl Container13 Prompt: DIP Joint
  MC. R : PMIOPort  Side=Left
  MCP Joint : PMIOPort  Port=2  Side=Left
  PIP Joint : PMIOPort  Port=3  Side=Left
  DIP Joint : PMIOPort  Port=4  Side=Left
  connections:
  PIP Joint/RConn1 -- Digit Links and Joints/LConn10
  Digit Links and Joints/LConn15 -- MCP Joint/RConn1
  MC. R/RConn1 -- Digit Links and Joints/LConn20
  DIP Joint/RConn1 -- Digit Links and Joints/LConn5

== system mesh_assembly/Digit IV ==
  note: MC. == Metacarpal
  Digit Links and Joints : Subsystem  AncestorBlock=mechanics_model_library/Digit  mask{links_density=dnm.link_density, distal_phalanx=knm.d4.distal_phalanx.file_name, distal_phalanx_base=knm.d4.distal_phalanx.base_transform, distal_phalanx_dip_joint=knm.d4.distal_phalanx.dip_joint_transform, distal_phalanx_head=knm.d4.distal_phalanx.head_transform, middle_phalanx=knm.d4.middle_phalanx.file_name, middle_phalanx_base=knm.d4.middle_phalanx.base_transform, middle_phalanx_pip_joint=knm.d4.middle_phalanx.pip_joint_transform, middle_phalanx_head=knm.d4.middle_phalanx.head_transform, middle_phalanx_dip_joint=knm.d4.middle_phalanx.dip_joint_transform, proximal_phalanx=knm.d4.proximal_phalanx.file_name, proximal_phalanx_base=knm.d4.proximal_phalanx.base_transform, proximal_phalanx_mcp_joint=knm.d4.proximal_phalanx.mcp_joint_transform, proximal_phalanx_head=knm.d4.proximal_phalanx.head_transform, proximal_phalanx_pip_joint=knm.d4.proximal_phalanx.pip_joint_transform, metacarpal=knm.d4.metacarpal.file_name, metacarpal_base=knm.d4.metacarpal.base_transform, metacarpal_cm_joint=knm.d4.metacarpal.cm_joint_transform, metacarpal_head=knm.d4.metacarpal.head_transform, metacarpal_mcp_joint=knm.d4.metacarpal.mcp_joint_transform, mcp_viz_radius=viz.d4.mcp_joint.radius, mcp_viz_color=viz.d4.mcp_joint.color, mcp_viz_opacity=viz.d4.mcp_joint.opacity, pip_viz_radius=viz.d4.pip_joint.radius, pip_viz_length=viz.d4.pip_joint.length, pip_viz_thickness=viz.d4.pip_joint.thickness, pip_viz_color=viz.d4.pip_joint.color, pip_viz_opacity=viz.d4.pip_joint.opacity, dip_viz_radius=viz.d4.dip_joint.radius, dip_viz_length=viz.d4.dip_joint.length, dip_viz_thickness=viz.d4.dip_joint.thickness, dip_viz_color=viz.d4.dip_joint.color, dip_viz_opacity=viz.d4.dip_joint.opacity}
      mask prompts: links_density "Density [Kg/(m^3)]"; distal_phalanx "File Name"; distal_phalanx_base "Base Transform (Translation [m], Rotation: X-Y-Z [deg])"; distal_phalanx_dip_joint "DIP Joint Transform (Translation, Rotation)"; distal_phalanx_head "Head Transform (Translation, Rotation)"; middle_phalanx "File Name"; middle_phalanx_base "Base Transform"; middle_phalanx_pip_joint "PIP Joint Transform"; middle_phalanx_head "Head Transform"; middle_phalanx_dip_joint "DIP Joint Transform"; proximal_phalanx "File Name"; proximal_phalanx_base "Base Transform"; proximal_phalanx_mcp_joint "MCP Joint Transform"; proximal_phalanx_head "Head Transform"; proximal_phalanx_pip_joint "PIP Joint Transform"; metacarpal "File Name"; metacarpal_base "Base Transform"; metacarpal_cm_joint "CM Joint Transform"; metacarpal_head "Head Transform"; metacarpal_mcp_joint "MCP Joint Transform"; mcp_viz_radius "Radius [m]"; mcp_viz_color "Color (RGB - Range [0, 1])"; mcp_viz_opacity "Opacity (Range [0, 1])"; pip_viz_radius "Radius [m]"; pip_viz_length "Length [m]"; pip_viz_thickness "Thickness [m]"; pip_viz_color "Color (RGB - Range [0, 1])"; pip_viz_opacity "Opacity (Range [0, 1])"; dip_viz_radius "Radius [m]"; dip_viz_length "Length [m]"; dip_viz_thickness "Thickness [m]"; dip_viz_color "Color (RGB - Range [0, 1])"; dip_viz_opacity "Opacity (Range [0, 1])"
      mask DialogControl DescGroupVar Prompt: Digit Subsystem
      mask DialogControl DescTextVar Prompt: This subsystem encapsulates the bones and joints that makes up digits II - V. Metacarpal bone, Proximal, Middle and Distal Phalanxes; MCP, PIP and DIP Joints.
      mask DialogControl Links Prompt: Links
      mask DialogControl Distal_Phalanx Prompt: Distal Phalanx
      mask DialogControl Middle_Phalanx Prompt: Middle Phalanx
      mask DialogControl Proximal_Phalanx Prompt: Proximal Phalanx
      mask DialogControl Metacarpal Prompt: Metacarpal
      mask DialogControl Container10 Prompt: Visualization
      mask DialogControl Container11 Prompt: MCP Joint
      mask DialogControl Container12 Prompt: PIP Joint
      mask DialogControl Container13 Prompt: DIP Joint
  Ligament Transform : sm_lib/Frames and Transforms/Rigid Transform  TranslationMethod=StandardAxis  TranslationStandardOffset=viz.d4.mcp_joint.radius  TranslationLengthUnit=m  TranslationStandardAxis=+Y  TranslationCartesianOffset=[0 0 0]  TranslationROffset=0  TranslationROffsetUnits=m  TranslationZOffset=0  TranslationZOffsetUnits=m  TranslationThetaOffset=0  TranslationThetaOffsetUnits=deg  RotationMethod=None  RotationAngleUnits=deg  RotationStandardAxis=+Z  RotationAngle=0.0  RotationArbitraryAxis=[0 0 1]  FollAlignAxisA=+X  BaseAlignAxisA=+Y  FollAlignAxisB=+Y  BaseAlignAxisB=+Z  RotationSequenceAxes=FollowerAxes  RotationSequence=XYX  RotationSequenceAngles=[0 0 0]  RotationSequenceAnglesUnits=deg  RotationMatrix=[1 0 0; 0 1 0; 0 0 1]
  Contraint Ligament : PMIOPort  Side=Left
  MCP Joint : PMIOPort  Port=2  Side=Left
  PIP Joint : PMIOPort  Port=3  Side=Left
  DIP Joint : PMIOPort  Port=4  Side=Left
  MC. R : PMIOPort  Port=5  Side=Left
  connections:
  Contraint Ligament/RConn1 -- Ligament Transform/RConn1
  DIP Joint/RConn1 -- Digit Links and Joints/LConn5
  Ligament Transform/LConn1 -- Digit Links and Joints/LConn15 -- MCP Joint/RConn1
  PIP Joint/RConn1 -- Digit Links and Joints/LConn10
  MC. R/RConn1 -- Digit Links and Joints/LConn20

== system mesh_assembly/Digit V ==
  note: MC. == Metacarpal
  Digit Links and Joints : Subsystem  AncestorBlock=mechanics_model_library/Digit  mask{links_density=dnm.link_density, distal_phalanx=knm.d5.distal_phalanx.file_name, distal_phalanx_base=knm.d5.distal_phalanx.base_transform, distal_phalanx_dip_joint=knm.d5.distal_phalanx.dip_joint_transform, distal_phalanx_head=knm.d5.distal_phalanx.head_transform, middle_phalanx=knm.d5.middle_phalanx.file_name, middle_phalanx_base=knm.d5.middle_phalanx.base_transform, middle_phalanx_pip_joint=knm.d5.middle_phalanx.pip_joint_transform, middle_phalanx_head=knm.d5.middle_phalanx.head_transform, middle_phalanx_dip_joint=knm.d5.middle_phalanx.dip_joint_transform, proximal_phalanx=knm.d5.proximal_phalanx.file_name, proximal_phalanx_base=knm.d5.proximal_phalanx.base_transform, proximal_phalanx_mcp_joint=knm.d5.proximal_phalanx.mcp_joint_transform, proximal_phalanx_head=knm.d5.proximal_phalanx.head_transform, proximal_phalanx_pip_joint=knm.d5.proximal_phalanx.pip_joint_transform, metacarpal=knm.d5.metacarpal.file_name, metacarpal_base=knm.d5.metacarpal.base_transform, metacarpal_cm_joint=knm.d5.metacarpal.cm_joint_transform, metacarpal_head=knm.d5.metacarpal.head_transform, metacarpal_mcp_joint=knm.d5.metacarpal.mcp_joint_transform, mcp_viz_radius=viz.d5.mcp_joint.radius, mcp_viz_color=viz.d5.mcp_joint.color, mcp_viz_opacity=viz.d5.mcp_joint.opacity, pip_viz_radius=viz.d5.pip_joint.radius, pip_viz_length=viz.d5.pip_joint.length, pip_viz_thickness=viz.d5.pip_joint.thickness, pip_viz_color=viz.d5.pip_joint.color, pip_viz_opacity=viz.d5.pip_joint.opacity, dip_viz_radius=viz.d5.dip_joint.radius, dip_viz_length=viz.d5.dip_joint.length, dip_viz_thickness=viz.d5.dip_joint.thickness, dip_viz_color=viz.d5.dip_joint.color, dip_viz_opacity=viz.d5.dip_joint.opacity}
      mask prompts: links_density "Density [Kg/(m^3)]"; distal_phalanx "File Name"; distal_phalanx_base "Base Transform (Translation [m], Rotation: X-Y-Z [deg])"; distal_phalanx_dip_joint "DIP Joint Transform (Translation, Rotation)"; distal_phalanx_head "Head Transform (Translation, Rotation)"; middle_phalanx "File Name"; middle_phalanx_base "Base Transform"; middle_phalanx_pip_joint "PIP Joint Transform"; middle_phalanx_head "Head Transform"; middle_phalanx_dip_joint "DIP Joint Transform"; proximal_phalanx "File Name"; proximal_phalanx_base "Base Transform"; proximal_phalanx_mcp_joint "MCP Joint Transform"; proximal_phalanx_head "Head Transform"; proximal_phalanx_pip_joint "PIP Joint Transform"; metacarpal "File Name"; metacarpal_base "Base Transform"; metacarpal_cm_joint "CM Joint Transform"; metacarpal_head "Head Transform"; metacarpal_mcp_joint "MCP Joint Transform"; mcp_viz_radius "Radius [m]"; mcp_viz_color "Color (RGB - Range [0, 1])"; mcp_viz_opacity "Opacity (Range [0, 1])"; pip_viz_radius "Radius [m]"; pip_viz_length "Length [m]"; pip_viz_thickness "Thickness [m]"; pip_viz_color "Color (RGB - Range [0, 1])"; pip_viz_opacity "Opacity (Range [0, 1])"; dip_viz_radius "Radius [m]"; dip_viz_length "Length [m]"; dip_viz_thickness "Thickness [m]"; dip_viz_color "Color (RGB - Range [0, 1])"; dip_viz_opacity "Opacity (Range [0, 1])"
      mask DialogControl DescGroupVar Prompt: Digit Subsystem
      mask DialogControl DescTextVar Prompt: This subsystem encapsulates the bones and joints that makes up digits II - V. Metacarpal bone, Proximal, Middle and Distal Phalanxes; MCP, PIP and DIP Joints.
      mask DialogControl Links Prompt: Links
      mask DialogControl Distal_Phalanx Prompt: Distal Phalanx
      mask DialogControl Middle_Phalanx Prompt: Middle Phalanx
      mask DialogControl Proximal_Phalanx Prompt: Proximal Phalanx
      mask DialogControl Metacarpal Prompt: Metacarpal
      mask DialogControl Container10 Prompt: Visualization
      mask DialogControl Container11 Prompt: MCP Joint
      mask DialogControl Container12 Prompt: PIP Joint
      mask DialogControl Container13 Prompt: DIP Joint
  Ligament Transform : sm_lib/Frames and Transforms/Rigid Transform  TranslationMethod=StandardAxis  TranslationStandardOffset=viz.d5.mcp_joint.radius  TranslationLengthUnit=m  TranslationStandardAxis=+Y  TranslationCartesianOffset=[0 0 0]  TranslationROffset=0  TranslationROffsetUnits=m  TranslationZOffset=0  TranslationZOffsetUnits=m  TranslationThetaOffset=0  TranslationThetaOffsetUnits=deg  RotationMethod=None  RotationAngleUnits=deg  RotationStandardAxis=+Z  RotationAngle=0.0  RotationArbitraryAxis=[0 0 1]  FollAlignAxisA=+X  BaseAlignAxisA=+Y  FollAlignAxisB=+Y  BaseAlignAxisB=+Z  RotationSequenceAxes=FollowerAxes  RotationSequence=XYX  RotationSequenceAngles=[0 0 0]  RotationSequenceAnglesUnits=deg  RotationMatrix=[1 0 0; 0 1 0; 0 0 1]
  MCP Joint : PMIOPort  Side=Left
  PIP Joint : PMIOPort  Port=2  Side=Left
  DIP Joint : PMIOPort  Port=3  Side=Left
  CM Joint : PMIOPort  Port=4  Side=Left
  Contraint Ligament : PMIOPort  Port=5  Side=Right
  connections:
  Contraint Ligament/RConn1 -- Ligament Transform/RConn1
  DIP Joint/RConn1 -- Digit Links and Joints/LConn5
  Ligament Transform/LConn1 -- Digit Links and Joints/LConn15 -- MCP Joint/RConn1
  PIP Joint/RConn1 -- Digit Links and Joints/LConn10
  CM Joint/RConn1 -- Digit Links and Joints/LConn19
